simulink model "sim1"  (R2021b)
settings: Solver=VariableStepAuto  StartTime=0.0  StopTime=10  RelTol=1e-3
settings Model: Creator=WIEiK-STUDENT  LastModifiedBy=me
settings SolverCC: AlgebraicLoopSolver=TrustRegion
settings DataIOCC: ReturnWorkspaceOutputs=off
settings DebuggingCC: SFMachineParentedDataDiag=warning  ArithmeticOperatorsInVariantConditions=warning
settings SFSimCC: CustomCodeUndefinedFunction=UseInterfaceOnly

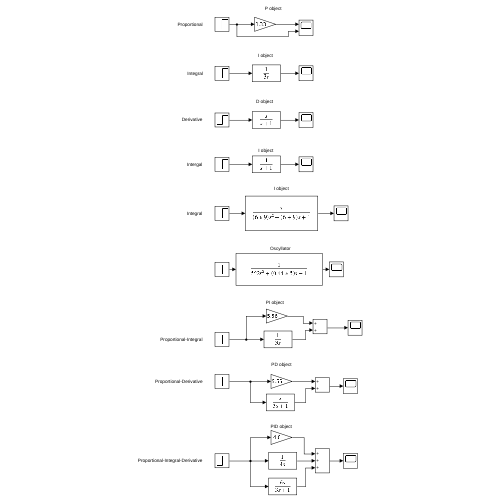
[thumbnail: Simulink's stored preview of the top-level diagram]
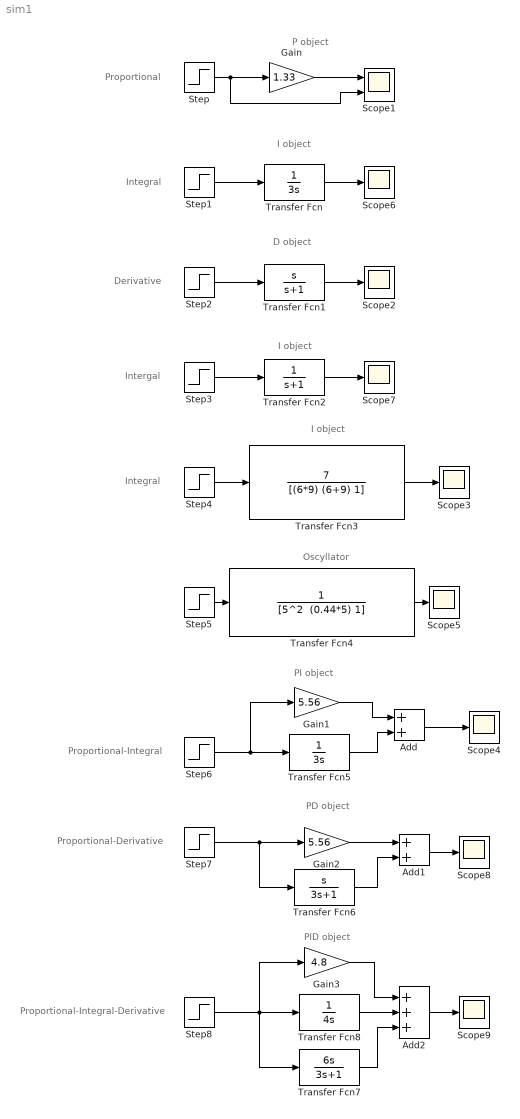
== system sim1 ==
  note: Integral
  note: Intergal
  note: Derivative
  note: Integral
  note: Proportional
  note: I object
  note: I object
  note: Proportional-Integral-Derivative
  note: Proportional-Derivative
  note: Proportional-Integral
  note: PD object
  note: PI object
  note: Oscyllator
  note: D object
  note: I object
  note: P object
  note: PID object
  Add : Sum
  Add1 : Sum
  Add2 : Sum  Inputs=+++
  Gain : Gain  Gain=1.33
  Gain1 : Gain  Gain=5.56
  Gain2 : Gain  Gain=5.56
  Gain3 : Gain  Gain=4.8
  Scope1 : Scope  NumInputPorts=2
  Scope{2..9} (8 alike) : Scope
  Step{,1..8} (9 alike) : Step  SampleTime=0
  Transfer Fcn : TransferFcn  Denominator=[3 0]
  Transfer Fcn1 : TransferFcn  Numerator=[1 0]  Denominator=[1 1]
  Transfer Fcn2 : TransferFcn  Denominator=[1 1]
  Transfer Fcn3 : TransferFcn  Numerator=[7]  Denominator=[(6*9) (6+9) 1]
  Transfer Fcn4 : TransferFcn  Denominator="[5^2  (0.44*5) 1]"
  Transfer Fcn5 : TransferFcn  Denominator=[3 0]
  Transfer Fcn6 : TransferFcn  Numerator=[1 0]  Denominator=[3 1]
  Transfer Fcn7 : TransferFcn  Numerator=[6 0]  Denominator=[3 1]
  Transfer Fcn8 : TransferFcn  Denominator=[4 0]
  wires:
  Step/1 -> Scope1/2, Gain/1
  Gain/1 -> Scope1/1
  Step1/1 -> Transfer Fcn/1
  Step2/1 -> Transfer Fcn1/1
  Step3/1 -> Transfer Fcn2/1
  Step4/1 -> Transfer Fcn3/1
  Step5/1 -> Transfer Fcn4/1
  Transfer Fcn4/1 -> Scope5/1
  Transfer Fcn/1 -> Scope6/1
  Transfer Fcn1/1 -> Scope2/1
  Transfer Fcn2/1 -> Scope7/1
  Transfer Fcn3/1 -> Scope3/1
  Step6/1 -> Gain1/1, Transfer Fcn5/1
  Transfer Fcn5/1 -> Add/2
  Gain1/1 -> Add/1
  Add/1 -> Scope4/1
  Add1/1 -> Scope8/1
  Transfer Fcn6/1 -> Add1/2
  Gain2/1 -> Add1/1
  Step7/1 -> Transfer Fcn6/1, Gain2/1
  Add2/1 -> Scope9/1
  Transfer Fcn7/1 -> Add2/3
  Step8/1 -> Transfer Fcn8/1, Transfer Fcn7/1, Gain3/1
  Gain3/1 -> Add2/1
  Transfer Fcn8/1 -> Add2/2
